simulink model "PendAndHeadingCtrlLQR"  (R2015b)
settings: Solver=VariableStepAuto  StartTime=0.0  StopTime=inf  RelTol=1e-3
undefined symbols (not defined in the file or in its folder): C_nuParams, D, D_nuParams, InitialPos, invM, invT, K2, K3, K4, K_lqr, Kd, Kp, pinvTr, ref, Tr
libraries: robotlib x11, realtime_pacer_lib x1
settings Model: Creator=saucer  LastModifiedBy=saucer

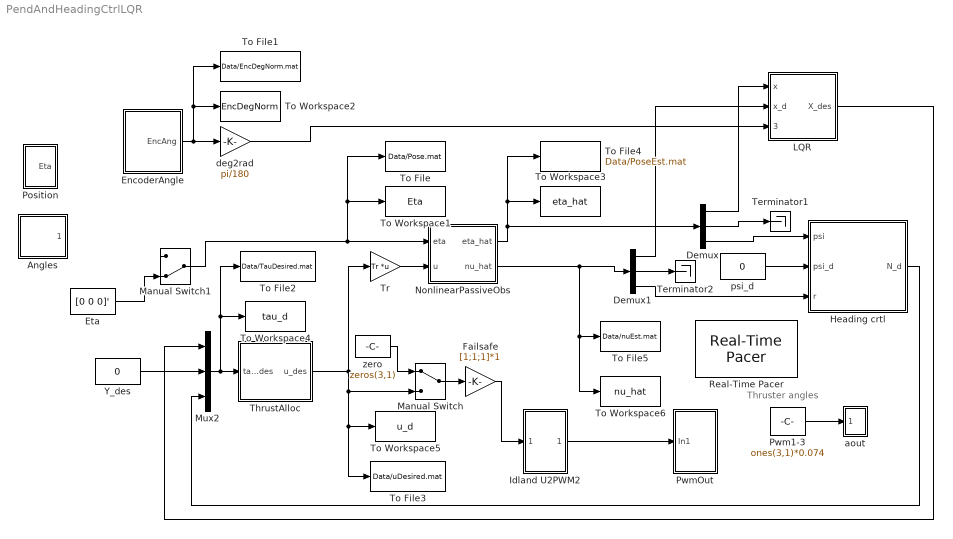
== system PendAndHeadingCtrlLQR ==
  note: Thruster angles
  Angles : Subsystem
  Demux : Demux  Outputs=3
  Demux1 : Demux  Outputs=3
  EncoderAngle : Subsystem
  Eta : Constant  Value=[0 0 0]'
  Failsafe : Gain  Gain=[1;1;1]*1
  Heading crtl : Subsystem
  Idland U2PWM2 : Subsystem
  LQR : Subsystem
  Manual Switch : ManualSwitch
  Manual Switch1 : ManualSwitch  CurrentSetting=0
  Mux2 : Mux  Inputs=3
  NonlinearPassiveObs : Subsystem
  Position : Subsystem
  Pwm1-3 : Constant  Value=ones(3,1)*0.074
  PwmOut : Subsystem
  Real-Time Pacer : realtime_pacer_lib/Real-Time Pacer  simTimePerRealTime=1
  Terminator1 : Terminator
  Terminator2 : Terminator
  ThrustAlloc : Subsystem
  To File : ToFile  Filename=Data/Pose.mat  MatrixName=Eta_measured  SaveFormat=Timeseries
  To File1 : ToFile  Filename=Data/EncDegNorm.mat  MatrixName=EncDegNorm  SaveFormat=Timeseries
  To File2 : ToFile  Filename=Data/TauDesired.mat  MatrixName=tau_d  SaveFormat=Timeseries
  To File3 : ToFile  Filename=Data/uDesired.mat  MatrixName=u_d  SaveFormat=Timeseries
  To File4 : ToFile  Filename=Data/PoseEst.mat  MatrixName=eta_hat  SaveFormat=Timeseries
  To File5 : ToFile  Filename=Data/nuEst.mat  MatrixName=nu_hat  SaveFormat=Timeseries
  To Workspace1 : ToWorkspace  VariableName=Eta  SaveFormat=Timeseries  SampleTime=-1
  To Workspace2 : ToWorkspace  VariableName=EncDegNorm  SaveFormat=Timeseries  SampleTime=-1
  To Workspace3 : ToWorkspace  VariableName=eta_hat  SaveFormat=Timeseries  SampleTime=-1
  To Workspace4 : ToWorkspace  VariableName=tau_d  SaveFormat=Timeseries  SampleTime=-1
  To Workspace5 : ToWorkspace  VariableName=u_d  SaveFormat=Timeseries  SampleTime=-1
  To Workspace6 : ToWorkspace  VariableName=nu_hat  SaveFormat=Timeseries  SampleTime=-1
  Tr : Gain  Gain=Tr  Multiplication=Matrix(K*u)
  Y_des : Constant  Value=0
  aout : Subsystem
  deg2rad : Gain  Gain=pi/180
  psi_d : Constant  Value=0
  zero : Constant  Value=zeros(3,1)
  wires:
  Pwm1-3/1 -> aout/1(In1)
  ThrustAlloc/1(u_des) -> Manual Switch/2, To File3/1, To Workspace5/1, Tr/1
  Idland U2PWM2/1(Out1) -> PwmOut/1(In1)
  Mux2/1 -> To File2/1, To Workspace4/1, ThrustAlloc/1(tau_des)
  EncoderAngle/1(EncAng) -> deg2rad/1, To Workspace2/1, To File1/1
  Tr/1 -> NonlinearPassiveObs/2(u)
  NonlinearPassiveObs/1(eta_hat) -> Demux/1, To Workspace3/1, To File4/1
  Demux/3 -> Heading crtl/1(psi)
  Demux1/3 -> Heading crtl/3(r)
  psi_d/1 -> Heading crtl/2(psi_d)
  Y_des/1 -> Mux2/2
  Failsafe/1 -> Idland U2PWM2/1(In1)
  Demux/2 -> Terminator1/1
  Demux1/2 -> Terminator2/1
  NonlinearPassiveObs/2(nu_hat) -> To Workspace6/1, To File5/1, Demux1/1
  Heading crtl/1(N_d) -> Mux2/3
  deg2rad/1 -> LQR/3(theta_1)
  LQR/1(X_des) -> Mux2/1
  Demux/1 -> LQR/1(x)
  Demux1/1 -> LQR/2(x_d)
  Manual Switch/1 -> Failsafe/1
  zero/1 -> Manual Switch/1
  ? -> Manual Switch1/1
  Manual Switch1/1 -> To File/1, To Workspace1/1, NonlinearPassiveObs/1(eta)
  Eta/1 -> Manual Switch1/2

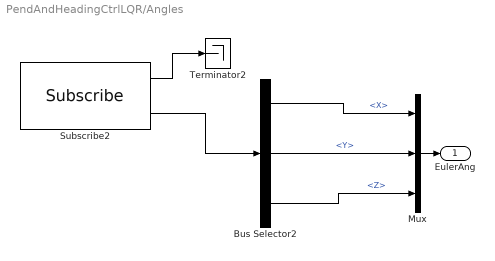
== system PendAndHeadingCtrlLQR/Angles ==
  Bus Selector2 : BusSelector  OutputSignals=X,Y,Z
  Mux : Mux  Inputs=3
  Subscribe2 : robotlib/Subscribe  SourceLibraryInfo=This block requires Robotics System Toolbox  topicSource=Select from ROS network  topic=/EulerAng  messageType=geometry_msgs/Vector3  sampleTime=-1  messageQueueLength=1
  Terminator2 : Terminator
  EulerAng : Outport
  wires:
  Bus Selector2/3 -> Mux/3  "<Z>"
  Bus Selector2/2 -> Mux/2  "<Y>"
  Subscribe2/1 -> Terminator2/1
  Mux/1 -> EulerAng/1
  Subscribe2/2 -> Bus Selector2/1
  Bus Selector2/1 -> Mux/1  "<X>"

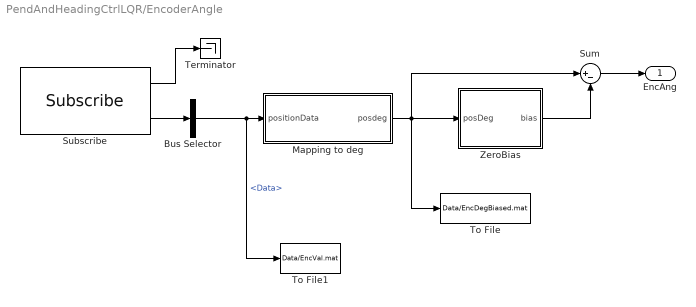
== system PendAndHeadingCtrlLQR/EncoderAngle ==
  Bus Selector : BusSelector  OutputSignals=Data
  Mapping to deg : MATLAB Function  TreatAsAtomicUnit=on
  Subscribe : robotlib/Subscribe  SourceLibraryInfo=This block requires Robotics System Toolbox  topicSource=Select from ROS network  topic=/encoder  messageType=std_msgs/Int64  sampleTime=-1  messageQueueLength=1
  Sum : Sum  Inputs=|+-
  Terminator : Terminator
  To File : ToFile  Filename=Data/EncDegBiased.mat  MatrixName=EncDegBias  SaveFormat=Timeseries
  To File1 : ToFile  Filename=Data/EncVal.mat  MatrixName=EncVal  SaveFormat=Timeseries
  ZeroBias : Subsystem
  EncAng : Outport
  wires:
  Subscribe/1 -> Terminator/1
  ZeroBias/1(bias) -> Sum/2
  Subscribe/2 -> Bus Selector/1
  Bus Selector/1 -> To File1/1, Mapping to deg/1(positionData)  "<Data>"
  Mapping to deg/1(posdeg) -> To File/1, ZeroBias/1(posDeg), Sum/1
  Sum/1 -> EncAng/1

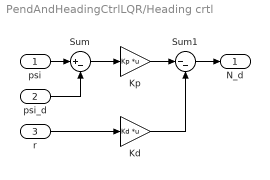
== system PendAndHeadingCtrlLQR/Heading crtl ==
  psi : Inport
  psi_d : Inport  Port=2
  r : Inport  Port=3
  Kd : Gain  Gain=Kd  Multiplication=Matrix(K*u)
  Kp : Gain  Gain=Kp  Multiplication=Matrix(K*u)
  Sum : Sum  Inputs=|+-
  Sum1 : Sum  Inputs=|--
  N_d : Outport
  wires:
  psi/1 -> Sum/1
  psi_d/1 -> Sum/2
  Sum/1 -> Kp/1
  r/1 -> Kd/1
  Kp/1 -> Sum1/1
  Kd/1 -> Sum1/2
  Sum1/1 -> N_d/1

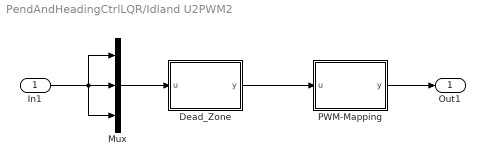
== system PendAndHeadingCtrlLQR/Idland U2PWM2 ==
  In1 : Inport
  Dead_Zone : MATLAB Function  TreatAsAtomicUnit=on
  Mux : Mux  Inputs=3
  PWM-Mapping : MATLAB Function  TreatAsAtomicUnit=on
  Out1 : Outport
  wires:
  Dead_Zone/1(y) -> PWM-Mapping/1(u)
  In1/1 -> Mux/1, Mux/2, Mux/3
  Mux/1 -> Dead_Zone/1(u)
  PWM-Mapping/1(y) -> Out1/1

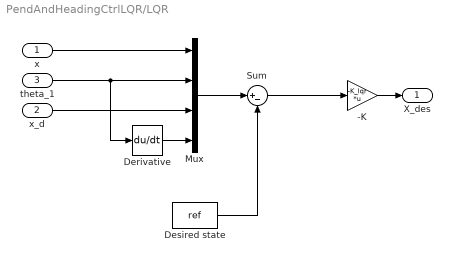
== system PendAndHeadingCtrlLQR/LQR ==
  x : Inport
  x_d : Inport  Port=2
  theta_1 : Inport  Port=3
  -K : Gain  Gain=-K_lqr  Multiplication=Matrix(K*u)
  Derivative : Derivative
  Desired state : Constant  Value=ref
  Mux : Mux
  Sum : Sum  Inputs=|+-
  X_des : Outport
  wires:
  Desired state/1 -> Sum/2
  theta_1/1 -> Mux/2, Derivative/1
  Derivative/1 -> Mux/4
  x/1 -> Mux/1
  Mux/1 -> Sum/1
  -K/1 -> X_des/1
  Sum/1 -> -K/1
  x_d/1 -> Mux/3

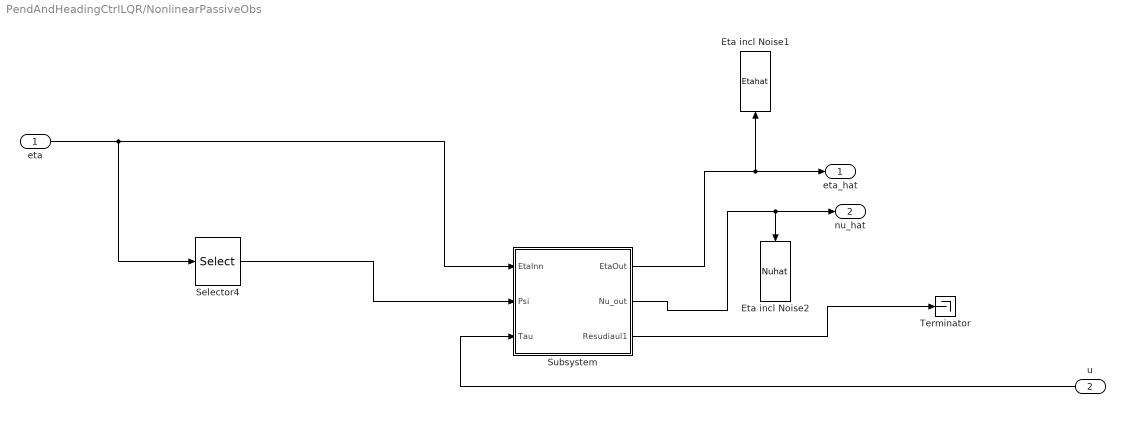
== system PendAndHeadingCtrlLQR/NonlinearPassiveObs ==
  eta : Inport
  u : Inport  Port=2
  Eta incl Noise1 : ToWorkspace  VariableName=Etahat  SaveFormat=Timeseries  SampleTime=-1
  Eta incl Noise2 : ToWorkspace  VariableName=Nuhat  SaveFormat=Timeseries  SampleTime=-1
  Selector4 : Selector  InputPortWidth=3  IndexOptions=Index vector (dialog)  Indices=3  OutputSizes=1
  Subsystem : Subsystem
  Terminator : Terminator
  eta_hat : Outport
  nu_hat : Outport  Port=2
  wires:
  Subsystem/3("Resudiaul1 ") -> Terminator/1
  eta/1 -> Selector4/1, Subsystem/1(EtaInn)
  Selector4/1 -> Subsystem/2(Psi)
  u/1 -> Subsystem/3("Tau ")
  Subsystem/2("Nu_out ") -> Eta incl Noise2/1, nu_hat/1
  Subsystem/1("EtaOut ") -> Eta incl Noise1/1, eta_hat/1

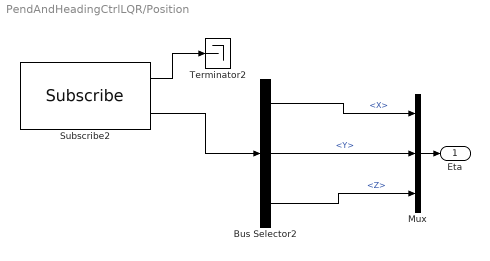
== system PendAndHeadingCtrlLQR/Position ==
  Bus Selector2 : BusSelector  OutputSignals=X,Y,Z
  Mux : Mux  Inputs=3
  Subscribe2 : robotlib/Subscribe  SourceLibraryInfo=This block requires Robotics System Toolbox  topicSource=Select from ROS network  topic=/Eta  messageType=geometry_msgs/Vector3  sampleTime=-1  messageQueueLength=1
  Terminator2 : Terminator
  Eta : Outport
  wires:
  Bus Selector2/1 -> Mux/1  "<X>"
  Subscribe2/2 -> Bus Selector2/1
  Mux/1 -> Eta/1
  Subscribe2/1 -> Terminator2/1
  Bus Selector2/2 -> Mux/2  "<Y>"
  Bus Selector2/3 -> Mux/3  "<Z>"

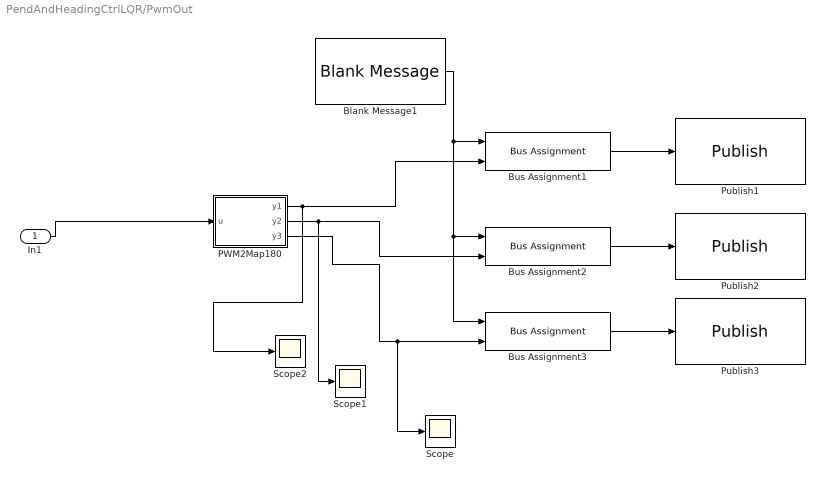
== system PendAndHeadingCtrlLQR/PwmOut ==
  In1 : Inport
  Blank Message1 : robotlib/Blank Message  SourceLibraryInfo=This block requires Robotics System Toolbox  messageType=std_msgs/UInt16  SampleTime=inf
  Bus Assignment1 : BusAssignment  AssignedSignals=Data
  Bus Assignment2 : BusAssignment  AssignedSignals=Data
  Bus Assignment3 : BusAssignment  AssignedSignals=Data
  "PWM2Map180 " : MATLAB Function  TreatAsAtomicUnit=on
  Publish1 : robotlib/Publish  SourceLibraryInfo=This block requires Robotics System Toolbox  topicSource=Specify your own  topic=/Thrust1  messageType=std_msgs/UInt16  messageQueueLength=1
  Publish2 : robotlib/Publish  SourceLibraryInfo=This block requires Robotics System Toolbox  topicSource=Specify your own  topic=/Thrust2  messageType=std_msgs/UInt16  messageQueueLength=1
  Publish3 : robotlib/Publish  SourceLibraryInfo=This block requires Robotics System Toolbox  topicSource=Specify your own  topic=/Thrust3  messageType=std_msgs/UInt16  messageQueueLength=1
  Scope : Scope
  Scope1 : Scope
  Scope2 : Scope
  wires:
  Bus Assignment3/1 -> Publish3/1
  "PWM2Map180 "/2(y2) -> Bus Assignment2/2, Scope1/1
  Bus Assignment1/1 -> Publish1/1
  Blank Message1/1 -> Bus Assignment3/1, Bus Assignment2/1, Bus Assignment1/1
  In1/1 -> "PWM2Map180 "/1(u)
  "PWM2Map180 "/3(y3) -> Scope/1, Bus Assignment3/2
  "PWM2Map180 "/1(y1) -> Scope2/1, Bus Assignment1/2
  Bus Assignment2/1 -> Publish2/1

== system PendAndHeadingCtrlLQR/ThrustAlloc ==
  tau_des : Inport
  pinvTr : Gain  Gain=pinvTr  Multiplication=Matrix(K*u)
  u_des : Outport
  wires:
  pinvTr/1 -> u_des/1
  tau_des/1 -> pinvTr/1

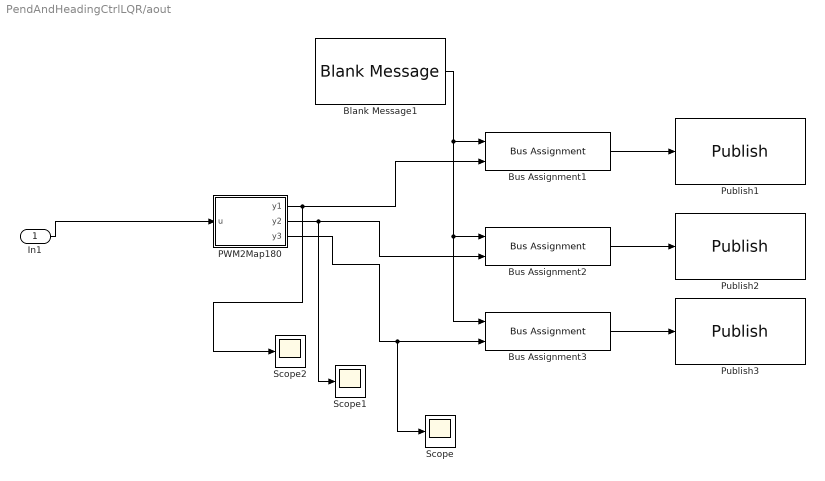
== system PendAndHeadingCtrlLQR/aout ==
  In1 : Inport
  Blank Message1 : robotlib/Blank Message  SourceLibraryInfo=This block requires Robotics System Toolbox  messageType=std_msgs/UInt16  SampleTime=inf
  Bus Assignment1 : BusAssignment  AssignedSignals=Data
  Bus Assignment2 : BusAssignment  AssignedSignals=Data
  Bus Assignment3 : BusAssignment  AssignedSignals=Data
  "PWM2Map180 " : MATLAB Function  TreatAsAtomicUnit=on
  Publish1 : robotlib/Publish  SourceLibraryInfo=This block requires Robotics System Toolbox  topicSource=Specify your own  topic=/a1  messageType=std_msgs/UInt16  messageQueueLength=1
  Publish2 : robotlib/Publish  SourceLibraryInfo=This block requires Robotics System Toolbox  topicSource=Specify your own  topic=/a2  messageType=std_msgs/UInt16  messageQueueLength=1
  Publish3 : robotlib/Publish  SourceLibraryInfo=This block requires Robotics System Toolbox  topicSource=Specify your own  topic=/a3  messageType=std_msgs/UInt16  messageQueueLength=1
  Scope : Scope
  Scope1 : Scope
  Scope2 : Scope
  wires:
  Bus Assignment2/1 -> Publish2/1
  "PWM2Map180 "/1(y1) -> Bus Assignment1/2, Scope2/1
  "PWM2Map180 "/3(y3) -> Bus Assignment3/2, Scope/1
  In1/1 -> "PWM2Map180 "/1(u)
  Blank Message1/1 -> Bus Assignment1/1, Bus Assignment2/1, Bus Assignment3/1
  Bus Assignment1/1 -> Publish1/1
  "PWM2Map180 "/2(y2) -> Scope1/1, Bus Assignment2/2
  Bus Assignment3/1 -> Publish3/1

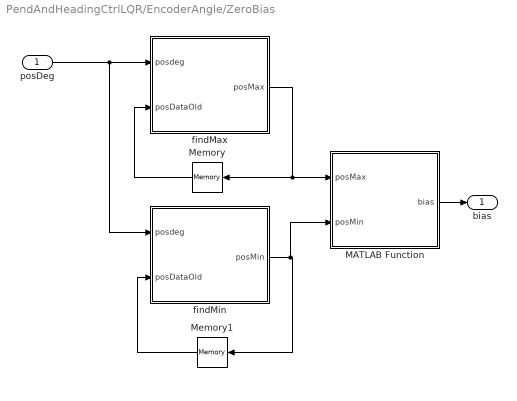
== system PendAndHeadingCtrlLQR/EncoderAngle/ZeroBias ==
  posDeg : Inport
  MATLAB Function : MATLAB Function  TreatAsAtomicUnit=on
  Memory : Memory  X0=-360
  Memory1 : Memory  X0=360
  findMax : MATLAB Function  TreatAsAtomicUnit=on
  findMin : MATLAB Function  TreatAsAtomicUnit=on
  bias : Outport
  wires:
  findMax/1(posMax) -> Memory/1, MATLAB Function/1(posMax)
  Memory/1 -> findMax/2(posDataOld)
  Memory1/1 -> findMin/2(posDataOld)
  findMin/1(posMin) -> MATLAB Function/2(posMin), Memory1/1
  MATLAB Function/1(bias) -> bias/1
  posDeg/1 -> findMin/1(posdeg), findMax/1(posdeg)

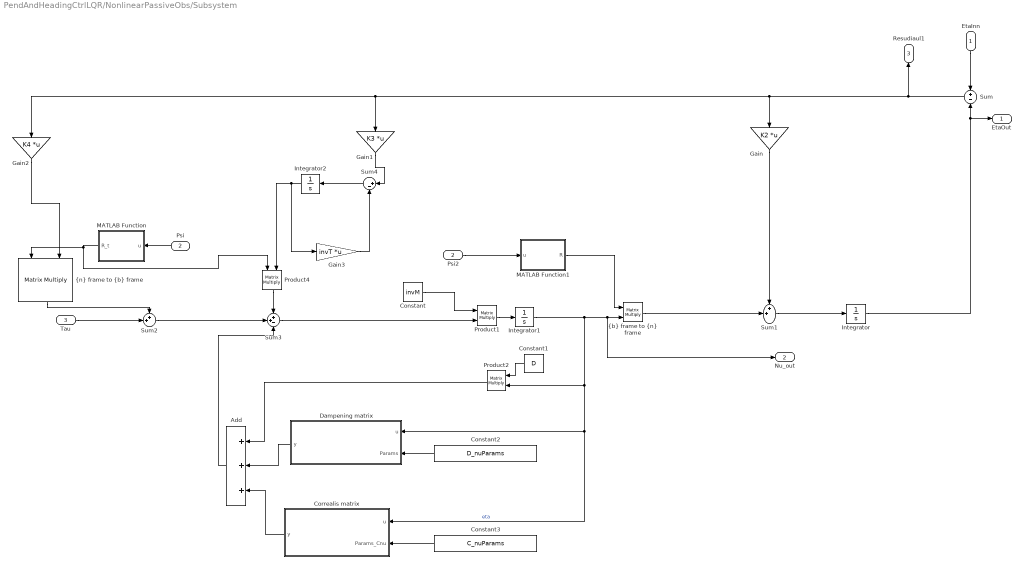
== system PendAndHeadingCtrlLQR/NonlinearPassiveObs/Subsystem ==
  EtaInn : Inport
  Psi : Inport  Port=2
  "Tau " : Inport  Port=3
  Add : Sum  Inputs=+++
  Constant : Constant  Value=invM
  Constant1 : Constant  Value=D
  Constant2 : Constant  Value=D_nuParams
  Constant3 : Constant  Value=C_nuParams
  Correalis matrix : MATLAB Function  TreatAsAtomicUnit=on
  Dampening matrix : MATLAB Function  TreatAsAtomicUnit=on
  Gain : Gain  Gain=K2  Multiplication=Matrix(K*u)
  Gain1 : Gain  Gain=K3  Multiplication=Matrix(K*u)
  Gain2 : Gain  Gain=K4  Multiplication=Matrix(K*u)
  Gain3 : Gain  Gain=invT  Multiplication=Matrix(K*u)
  Integrator : Integrator  InitialCondition=InitialPos
  Integrator1 : Integrator
  Integrator2 : Integrator  InitialCondition=[0;0;0]
  MATLAB Function : MATLAB Function  TreatAsAtomicUnit=on
  MATLAB Function1 : MATLAB Function  TreatAsAtomicUnit=on
  Product1 : Product  Multiplication=Matrix(*)
  Product2 : Product  Multiplication=Matrix(*)
  Product4 : Product  Multiplication=Matrix(*)
  Psi2 : InportShadow  Port=2
  Sum : Sum  Inputs=+|-
  Sum1 : Sum  Inputs=++|
  Sum2 : Sum  Inputs=++|
  Sum3 : Sum  Inputs=++-
  Sum4 : Sum  Inputs=|+-
  "{b} frame to {n} frame" : Product  Multiplication=Matrix(*)
  "{n} frame to {b} frame" : Product  Multiplication=Matrix(*)
  "EtaOut " : Outport
  "Nu_out " : Outport  Port=2
  "Resudiaul1 " : Outport  Port=3
  wires:
  Add/1 -> Sum3/3
  Correalis matrix/1(y) -> Add/3
  Dampening matrix/1(y) -> Add/2
  Product2/1 -> Add/1
  Integrator1/1 -> Product2/2, Dampening matrix/1(u), Correalis matrix/1(u), "Nu_out "/1, "{b} frame to {n} frame"/2  "eta"
  Constant3/1 -> Correalis matrix/2(Params_Cnu)
  Constant2/1 -> Dampening matrix/2(Params)
  Gain2/1 -> "{n} frame to {b} frame"/2
  EtaInn/1 -> Sum/1
  Sum/1 -> "Resudiaul1 "/1, Gain2/1, Gain1/1, Gain/1
  Gain/1 -> Sum1/1
  Sum1/1 -> Integrator/1
  Integrator/1 -> Sum/2, "EtaOut "/1
  Psi/1 -> MATLAB Function/1(u)
  "{n} frame to {b} frame"/1 -> Sum2/1
  "Tau "/1 -> Sum2/2
  Constant/1 -> Product1/1
  Product1/1 -> Integrator1/1
  Constant1/1 -> Product2/1
  Sum2/1 -> Sum3/2
  Sum3/1 -> Product1/2
  Psi2/1 -> MATLAB Function1/1(u)
  MATLAB Function1/1(R) -> "{b} frame to {n} frame"/1
  MATLAB Function/1(R_t) -> Product4/1, "{n} frame to {b} frame"/1
  "{b} frame to {n} frame"/1 -> Sum1/2
  Gain1/1 -> Sum4/1
  Sum4/1 -> Integrator2/1
  Integrator2/1 -> Product4/2, Gain3/1
  Gain3/1 -> Sum4/2
  Product4/1 -> Sum3/1

== matlab function PendAndHeadingCtrlLQR/EncoderAngle/Mapping to deg ==
  data: positionData input; posdeg output
function posdeg = val2deg(positionData)
%#codegen
puls = 2*2048; %2 channels x 2048 CPR
degpp = 360/puls; %Degrees pr. pulse.
% positionData = uint32(positionData); %Convert from double to uint32

%Convertion to signed data:
counterNBits = 12; %Bits in the encoder reading
signedThreshold = 2^(counterNBits-1); %Treshold for convertion to signed pos. values
signedData = positionData;
signedData(signedData > signedThreshold) = signedData(signedData > signedThreshold) - 2^counterNBits;

posdeg = signedData*degpp;

== matlab function PendAndHeadingCtrlLQR/PwmOut/PWM2Map180  ==
  data: u input; y1 output; y2 output; y3 output
function [y1,y2,y3] = fcn(u)
%#codegen
y1=uint16((u(1)-0.027)*180/0.093);
y2=uint16((u(2)-0.027)*180/0.093);
y3=uint16((u(3)-0.027)*180/0.093);

== matlab function PendAndHeadingCtrlLQR/EncoderAngle/ZeroBias/findMax ==
  data: posdeg input; posMax output; posDataOld input
function posMax = findMax(posdeg,posDataOld)
posMax = posDataOld;
if posdeg > posDataOld
    posMax = posdeg;
end

== matlab function PendAndHeadingCtrlLQR/EncoderAngle/ZeroBias/MATLAB Function ==
  data: posMax input; bias output; posMin input
function bias = normalRange(posMax,posMin)
range = posMax-posMin;
bias = posMin + range/2;

== matlab function PendAndHeadingCtrlLQR/aout/PWM2Map180  ==
  data: u input; y1 output; y2 output; y3 output
function [y1,y2,y3] = fcn(u)
%#codegen
y1=uint16((u(1)-0.027)*180/0.093);
y2=uint16((u(2)-0.027)*180/0.093);
y3=uint16((u(3)-0.027)*180/0.093);

== matlab function PendAndHeadingCtrlLQR/Idland U2PWM2/Dead_Zone ==
  data: u input; y output
function y = fcn(u)
%#codegen
y=[0 ;0 ;0];
for i=1:3
if (u(i)<-0.02);
    y(i)=u(i)*0.8-0.15;
elseif (u(i)>0.02)
    y(i)=u(i)*0.8+0.15;
end
end

== matlab function PendAndHeadingCtrlLQR/Idland U2PWM2/PWM-Mapping ==
  data: u input; y output
function y = fcn(u)
y=(u.*0.0255)+(0.0685);
end

== matlab function PendAndHeadingCtrlLQR/EncoderAngle/ZeroBias/findMin ==
  data: posdeg input; posMin output; posDataOld input
function posMin = findMin(posdeg,posDataOld)
posMin = posDataOld;
if posdeg < posDataOld
    posMin = posdeg;
end

== matlab function PendAndHeadingCtrlLQR/NonlinearPassiveObs/Subsystem/Correalis matrix ==
  data: u input; y output; Params_Cnu input
function y = fcn(u,Params_Cnu)
%#codegen
C=[0 Params_Cnu(2,1)*u(3) 0;-Params_Cnu(1,2)*u(3) 0 0;0 0 0];
y=C*u;

== matlab function PendAndHeadingCtrlLQR/NonlinearPassiveObs/Subsystem/Dampening matrix ==
  data: u input; y output; Params input
function y = fcn(u,Params)
%#codegen
Dnu=[Params(1,1)*abs(u(1)) 0 0;0 Params(2,2)*abs(u(2)) 0;0 0 0];
y=Dnu*u;

== matlab function PendAndHeadingCtrlLQR/NonlinearPassiveObs/Subsystem/MATLAB Function ==
  data: u input; R_t output
function R_t = fcn(u)
RotPhi=[cos(u) -sin(u) 0;sin(u) cos(u) 0 ;0 0 1];
R_t = RotPhi';
%R=[RotPhi(1:2,:);[0 0 0;0 0 0;0 0 0];RotPhi(3,:)]
end

== matlab function PendAndHeadingCtrlLQR/NonlinearPassiveObs/Subsystem/MATLAB Function1 ==
  data: u input; R output
function R = fcn(u)
RotPhi=[cos(u) -sin(u) 0;sin(u) cos(u) 0 ;0 0 1];
R = RotPhi;
end
